simulink model "KD_cl_harness_forthao"  (R2015a)
settings: Solver=ode45  StartTime=0  StopTime=50  FixedStep=0.01  MaxStep=0.005  RelTol=1e-4  AbsTol=1e-4
InitFcn:
  | load KD_const_coeffs_0624
  | load pexhat_stuff
  | load expcon
  | load thr_ff_map
values from neighbouring files (symbols this model uses):
  k1_table = [1 1 1 1 1 1 1 1 1 1 1 1 ... (42 elements, 6x7)]    [thr_ff_map.mat]
  k2_table = [1 1 1 1 1 1 1 1 1 1 1 1 ... (42 elements, 6x7)]    [thr_ff_map.mat]
undefined symbols (not defined in the file or in its folder): c_0, c_1, c_100, c_1000, c_10000, c_1000inv, c_100inv, c_1_int, c_1d2p4, c_1p7, c_4400inv, c_5500inv, c_80, c_90, c_cal_phi, c_compmap, c_ctok, c_fflow_max, c_fflow_min, c_filt, c_flowdiv, c_flowmin, c_flowmult, c_inf, c_km1d2k, c_mm3tokgpers, c_n1, c_p00001, c_p01, c_p016, c_p1429, c_p1e9, c_p4167, c_p4d1p4, c_p5401, c_p9, c_pincomp, c_ra, c_rair, c_Rby1000, c_roacorr, c_rpmtoradpers, c_svrthrottle1, c_svrthrottle2, c_svrthrottlearg, c_svrthrottlebeta, c_ta_max, c_ta_min, c_V, c_vnliftmax, c_vnliftmin, Coefs, const, const_exhat, eegr_map, egrr_delay_init, epim_map, eplufin_ff_map, expcon, invta ... (+15)
libraries: simulink x5
(part 4 of 5)

== system KD_cl_harness_forthao/ctrl_rb_explicit_20131031_v2/expcon/get_ctrl ==
  region : Inport
  u : Inport  Port=2
  calc_u_star : Subsystem
  u_star : Outport
  wires:
  calc_u_star/1(u_star) -> u_star/1
  u/1 -> calc_u_star/2(u)
  region/1 -> calc_u_star/1(region)

== system KD_cl_harness_forthao/ctrl_rb_explicit_20131031_v2/invert_flow/valve_inversion ==
  Ro_a : Inport
  pexhaust : Inport  Port=2
  pintake : Inport  Port=3
  uwegr : Inport  Port=4
  ne_rpm : Inport  Port=5
  Cal_phi1 : Subsystem
  Constant1 : Constant  Value=c_p4167  OutDataTypeStr=single
      settings: AttributesFormatString=%<Value>
  Constant3 : Constant  Value=c_p1429  OutDataTypeStr=single
      settings: AttributesFormatString=%<Value>
  Constant4 : Constant  Value=c_1  OutDataTypeStr=single
      settings: AttributesFormatString=%<Value>
  Constant5 : Constant  Value=c_p5401  OutDataTypeStr=single
      settings: AttributesFormatString=%<Value>
  Pm_by_Pex : Product  Inputs=*/  SaturateOnIntegerOverflow=on  RndMeth=Zero  InputSameDT=on  OutDataTypeStr=Inherit: Same as first input
  Relational Operator : RelationalOperator  Operator=>  OutDataTypeStr=boolean
      settings: AttributesFormatString=%<Operator>
  Saturation1 : Saturate  UpperLimit=c_1  LowerLimit=c_p4167
      settings: AttributesFormatString=%<LowerLimit>\n%<UpperLimit>
  Saturation2 : Saturate  UpperLimit=c_inf  LowerLimit=c_90
      settings: AttributesFormatString=%<LowerLimit>\n%<UpperLimit>
  Saturation3 : Saturate  UpperLimit=c_inf  LowerLimit=c_0
      settings: AttributesFormatString=%<LowerLimit>\n%<UpperLimit>
  Saturation4 : Saturate  UpperLimit=c_inf  LowerLimit=c_p00001
      settings: AttributesFormatString=%<LowerLimit>\n%<UpperLimit>
  Sqrt : Sqrt  AlgorithmType=Newton-Raphson  SaturateOnIntegerOverflow=on
  Sum : Sum  Inputs=|+-
  Sum1 : Sum  Inputs=|++
  Switch2 : Switch  Criteria=u2 ~= 0
      settings: AttributesFormatString=%<Criteria>
  correct flow1 : Product  Inputs=*/  SaturateOnIntegerOverflow=on  RndMeth=Zero  InputSameDT=on  OutDataTypeStr=Inherit: Same as first input
  correct flow2 : Product  Inputs=**  SaturateOnIntegerOverflow=on  RndMeth=Zero  InputSameDT=on  OutDataTypeStr=Inherit: Same as first input
  correct flow3 : Product  Inputs=**  SaturateOnIntegerOverflow=on  RndMeth=Zero  InputSameDT=on  OutDataTypeStr=Inherit: Same as first input
  correct flow4 : Product  Inputs=**  SaturateOnIntegerOverflow=on  RndMeth=Zero  InputSameDT=on  OutDataTypeStr=Inherit: Same as first input
  invert_svr_lut : Lookup2D  RowIndex=invtacols  ColumnIndex=invtarows  Table=invta  LookUpMeth=Interpolation-Use End Values
      settings: AttributesFormatString=%<LookUpMeth>\n%<RowIndex>\n%<ColumnIndex>
  togps : Gain  Gain=c_1000
      settings: AttributesFormatString=%<Gain>
  valve_angle : Outport
  wires:
  Sqrt/1 -> Switch2/1
  correct flow3/1 -> Saturation3/1
  correct flow2/1 -> Sum1/1
  Constant3/1 -> correct flow2/2
  Sum/1 -> correct flow2/1, correct flow3/1
  Constant4/1 -> Sum/1
  invert_svr_lut/1 -> valve_angle/1
  uwegr/1 -> togps/1
  Ro_a/1 -> Cal_phi1/2(Ro_a)
  pexhaust/1 -> [Pex], Saturation2/1
  pintake/1 -> Pm_by_Pex/1
  Pm_by_Pex/1 -> Saturation1/1, Relational Operator/1
  Saturation1/1 -> Sum1/2, Sum/2
  [Pex] -> Cal_phi1/1(Pa)
  Sum1/1 -> correct flow3/2
  Saturation2/1 -> Pm_by_Pex/2
  Saturation3/1 -> Sqrt/1
  Saturation4/1 -> correct flow1/2
  correct flow4/1 -> Saturation4/1
  Switch2/1 -> correct flow4/2
  Cal_phi1/1(phi) -> correct flow4/1
  togps/1 -> correct flow1/1
  Relational Operator/1 -> Switch2/2
  Constant5/1 -> Switch2/3
  Constant1/1 -> Relational Operator/2
  correct flow1/1 -> invert_svr_lut/2
  ne_rpm/1 -> invert_svr_lut/1

== system KD_cl_harness_forthao/ctrl_rb_explicit_20131031_v2/ntestimator/Throttle_Model ==
  TA_deg : Inport
  Ne_rpm : Inport  Port=2
  Pim_Pa : Inport  Port=3
  Tam_K : Inport  Port=4
  wegrthr : Inport  Port=5
  Air_Model_map_use : Subsystem
  Ra : Constant  Value=c_rair  OutDataTypeStr=single  SampleTime=sample_time
      settings: AttributesFormatString=%<Value>\n%<SampleTime>
  p_pre_throttle : Outport  OutDataTypeStr=single
  wires:
  TA_deg/1 -> Air_Model_map_use/1(TA_deg)
  Tam_K/1 -> Air_Model_map_use/4(Ta_K)
  Pim_Pa/1 -> Air_Model_map_use/3(Pim_Pa)
  Ra/1 -> Air_Model_map_use/5(R_a)
  Ne_rpm/1 -> Air_Model_map_use/2(Ne_rpm)
  wegrthr/1 -> Air_Model_map_use/6(wegrthr)
  Air_Model_map_use/1(p_pre_throttle) -> p_pre_throttle/1

== system KD_cl_harness_forthao/ctrl_rb_explicit_20131031_v2/ntestimator/custom_filter ==
  Input : Inport
  Delay1 : Delay  DelayLength=1  InitialCondition=0
  Product1 : Product  Inputs=**  RndMeth=Zero
  Product2 : Product  Inputs=**  RndMeth=Zero
  Saturation1 : Saturate  UpperLimit=1  LowerLimit=0
      settings: AttributesFormatString=%<LowerLimit>\n%<UpperLimit>
  Saturation4 : Saturate  UpperLimit=1  LowerLimit=0
      settings: AttributesFormatString=%<LowerLimit>\n%<UpperLimit>
  Sum1 : Sum  Inputs=+-|
  Sum11 : Sum  Inputs=++|
  filt : Constant  Value=c_filt  OutDataTypeStr=single  SampleTime=sample_time
      settings: AttributesFormatString=%<Value>\n%<SampleTime>
  filt1 : Constant  Value=c_filt  OutDataTypeStr=single  SampleTime=sample_time
      settings: AttributesFormatString=%<Value>\n%<SampleTime>
  one : Constant  OutDataTypeStr=single  SampleTime=sample_time
      settings: AttributesFormatString=%<Value>\n%<SampleTime>
  Output : Outport  OutDataTypeStr=single
  wires:
  Input/1 -> Product1/2
  Delay1/1 -> Product2/1
  filt/1 -> Saturation1/1
  Product2/1 -> Sum11/1
  Sum1/1 -> Product1/1
  filt1/1 -> Saturation4/1
  Saturation4/1 -> Sum1/2
  Saturation1/1 -> Product2/2
  Product1/1 -> Sum11/2
  one/1 -> Sum1/1
  Sum11/1 -> Output/1, Delay1/1

== system KD_cl_harness_forthao/ctrl_rb_explicit_20131031_v2/rpm1200testpattern/IfActionSubsystem ==
  Action Port : ActionPort  ActionType=then
  tp : Constant  Value=[150;50;150]  OutDataTypeStr=single  SampleTime=sample_time
      settings: AttributesFormatString=%<Value>\n%<SampleTime>
  Out1 : Outport  InitialOutput=[150;50;150]
  wires:
  tp/1 -> Out1/1

== system KD_cl_harness_forthao/ctrl_rb_explicit_20131031_v2/rpm1200testpattern/IfActionSubsystem1 ==
  Action Port : ActionPort  ActionType=elseif
  tp : Constant  Value=[150;50;150]  OutDataTypeStr=single  SampleTime=sample_time
      settings: AttributesFormatString=%<Value>\n%<SampleTime>
  Out1 : Outport  InitialOutput=[150;50;150]
  wires:
  tp/1 -> Out1/1

== system KD_cl_harness_forthao/ctrl_rb_explicit_20131031_v2/rpm1200testpattern/IfActionSubsystem10 ==
  Action Port : ActionPort  ActionType=elseif
  tp : Constant  Value=[150;50;150]  OutDataTypeStr=single  SampleTime=sample_time
      settings: AttributesFormatString=%<Value>\n%<SampleTime>
  Out1 : Outport  InitialOutput=[150;50;150]
  wires:
  tp/1 -> Out1/1

== system KD_cl_harness_forthao/ctrl_rb_explicit_20131031_v2/rpm1200testpattern/IfActionSubsystem11 ==
  Action Port : ActionPort  ActionType=elseif
  tp : Constant  Value=[150;50;150]  OutDataTypeStr=single  SampleTime=sample_time
      settings: AttributesFormatString=%<Value>\n%<SampleTime>
  Out1 : Outport  InitialOutput=[150;50;150]
  wires:
  tp/1 -> Out1/1

== system KD_cl_harness_forthao/ctrl_rb_explicit_20131031_v2/rpm1200testpattern/IfActionSubsystem12 ==
  Action Port : ActionPort  ActionType=elseif
  tp : Constant  Value=[150;50;150]  OutDataTypeStr=single  SampleTime=sample_time
      settings: AttributesFormatString=%<Value>\n%<SampleTime>
  Out1 : Outport  InitialOutput=[150;50;150]
  wires:
  tp/1 -> Out1/1

== system KD_cl_harness_forthao/ctrl_rb_explicit_20131031_v2/rpm1200testpattern/IfActionSubsystem13 ==
  Action Port : ActionPort  ActionType=elseif
  tp : Constant  Value=[150;50;150]  OutDataTypeStr=single  SampleTime=sample_time
      settings: AttributesFormatString=%<Value>\n%<SampleTime>
  Out1 : Outport  InitialOutput=[150;50;150]
  wires:
  tp/1 -> Out1/1

== system KD_cl_harness_forthao/ctrl_rb_explicit_20131031_v2/rpm1200testpattern/IfActionSubsystem14 ==
  Action Port : ActionPort  ActionType=elseif
  tp : Constant  Value=[150;50;150]  OutDataTypeStr=single  SampleTime=sample_time
      settings: AttributesFormatString=%<Value>\n%<SampleTime>
  Out1 : Outport  InitialOutput=[150;50;150]
  wires:
  tp/1 -> Out1/1

== system KD_cl_harness_forthao/ctrl_rb_explicit_20131031_v2/rpm1200testpattern/IfActionSubsystem15 ==
  Action Port : ActionPort  ActionType=elseif
  tp : Constant  Value=[150;20;150]  OutDataTypeStr=single  SampleTime=sample_time
      settings: AttributesFormatString=%<Value>\n%<SampleTime>
  Out1 : Outport  InitialOutput=[150;20;150]
  wires:
  tp/1 -> Out1/1

== system KD_cl_harness_forthao/ctrl_rb_explicit_20131031_v2/rpm1200testpattern/IfActionSubsystem16 ==
  Action Port : ActionPort  ActionType=elseif
  tp : Constant  Value=[150;5;150]  OutDataTypeStr=single  SampleTime=sample_time
      settings: AttributesFormatString=%<Value>\n%<SampleTime>
  Out1 : Outport  InitialOutput=[150;5;150]
  wires:
  tp/1 -> Out1/1

== system KD_cl_harness_forthao/ctrl_rb_explicit_20131031_v2/rpm1200testpattern/IfActionSubsystem17 ==
  Action Port : ActionPort  ActionType=elseif
  tp : Constant  Value=[150;15;150]  OutDataTypeStr=single  SampleTime=sample_time
      settings: AttributesFormatString=%<Value>\n%<SampleTime>
  Out1 : Outport  InitialOutput=[150;15;150]
  wires:
  tp/1 -> Out1/1

== system KD_cl_harness_forthao/ctrl_rb_explicit_20131031_v2/rpm1200testpattern/IfActionSubsystem18 ==
  Action Port : ActionPort  ActionType=elseif
  tp : Constant  Value=[130;20;150]  OutDataTypeStr=single  SampleTime=sample_time
      settings: AttributesFormatString=%<Value>\n%<SampleTime>
  Out1 : Outport  InitialOutput=[130;20;150]
  wires:
  tp/1 -> Out1/1

== system KD_cl_harness_forthao/ctrl_rb_explicit_20131031_v2/rpm1200testpattern/IfActionSubsystem19 ==
  Action Port : ActionPort  ActionType=elseif
  tp : Constant  Value=[130;20;115]  OutDataTypeStr=single  SampleTime=sample_time
      settings: AttributesFormatString=%<Value>\n%<SampleTime>
  Out1 : Outport  InitialOutput=[130;20;115]
  wires:
  tp/1 -> Out1/1

== system KD_cl_harness_forthao/ctrl_rb_explicit_20131031_v2/rpm1200testpattern/IfActionSubsystem2 ==
  Action Port : ActionPort  ActionType=elseif
  tp : Constant  Value=[150;50;150]  OutDataTypeStr=single  SampleTime=sample_time
      settings: AttributesFormatString=%<Value>\n%<SampleTime>
  Out1 : Outport  InitialOutput=[150;50;150]
  wires:
  tp/1 -> Out1/1

== system KD_cl_harness_forthao/ctrl_rb_explicit_20131031_v2/rpm1200testpattern/IfActionSubsystem20 ==
  Action Port : ActionPort  ActionType=elseif
  tp : Constant  Value=[130;20;110]  OutDataTypeStr=single  SampleTime=sample_time
      settings: AttributesFormatString=%<Value>\n%<SampleTime>
  Out1 : Outport  InitialOutput=[130;20;110]
  wires:
  tp/1 -> Out1/1

== system KD_cl_harness_forthao/ctrl_rb_explicit_20131031_v2/rpm1200testpattern/IfActionSubsystem21 ==
  Action Port : ActionPort  ActionType=elseif
  tp : Constant  Value=[130;20;105]  OutDataTypeStr=single  SampleTime=sample_time
      settings: AttributesFormatString=%<Value>\n%<SampleTime>
  Out1 : Outport  InitialOutput=[130;20;105]
  wires:
  tp/1 -> Out1/1

== system KD_cl_harness_forthao/ctrl_rb_explicit_20131031_v2/rpm1200testpattern/IfActionSubsystem22 ==
  Action Port : ActionPort  ActionType=elseif
  tp : Constant  Value=[130;0;105]  OutDataTypeStr=single  SampleTime=sample_time
      settings: AttributesFormatString=%<Value>\n%<SampleTime>
  Out1 : Outport  InitialOutput=[130;0;105]
  wires:
  tp/1 -> Out1/1

== system KD_cl_harness_forthao/ctrl_rb_explicit_20131031_v2/rpm1200testpattern/IfActionSubsystem23 ==
  Action Port : ActionPort  ActionType=elseif
  tp : Constant  Value=[130;0;110]  OutDataTypeStr=single  SampleTime=sample_time
      settings: AttributesFormatString=%<Value>\n%<SampleTime>
  Out1 : Outport  InitialOutput=[130;0;110]
  wires:
  tp/1 -> Out1/1

== system KD_cl_harness_forthao/ctrl_rb_explicit_20131031_v2/rpm1200testpattern/IfActionSubsystem24 ==
  Action Port : ActionPort  ActionType=elseif
  tp : Constant  Value=[150;3;150]  OutDataTypeStr=single  SampleTime=sample_time
      settings: AttributesFormatString=%<Value>\n%<SampleTime>
  Out1 : Outport  InitialOutput=[150;3;150]
  wires:
  tp/1 -> Out1/1

== system KD_cl_harness_forthao/ctrl_rb_explicit_20131031_v2/rpm1200testpattern/IfActionSubsystem25 ==
  Action Port : ActionPort  ActionType=elseif
  tp : Constant  Value=[150;10;150]  OutDataTypeStr=single  SampleTime=sample_time
      settings: AttributesFormatString=%<Value>\n%<SampleTime>
  Out1 : Outport  InitialOutput=[150;10;150]
  wires:
  tp/1 -> Out1/1

== system KD_cl_harness_forthao/ctrl_rb_explicit_20131031_v2/rpm1200testpattern/IfActionSubsystem26 ==
  Action Port : ActionPort  ActionType=elseif
  tp : Constant  Value=[150;20;150]  OutDataTypeStr=single  SampleTime=sample_time
      settings: AttributesFormatString=%<Value>\n%<SampleTime>
  Out1 : Outport  InitialOutput=[150;20;150]
  wires:
  tp/1 -> Out1/1

== system KD_cl_harness_forthao/ctrl_rb_explicit_20131031_v2/rpm1200testpattern/IfActionSubsystem27 ==
  Action Port : ActionPort  ActionType=elseif
  tp : Constant  Value=[150;20;150]  OutDataTypeStr=single  SampleTime=sample_time
      settings: AttributesFormatString=%<Value>\n%<SampleTime>
  Out1 : Outport  InitialOutput=[150;20;150]
  wires:
  tp/1 -> Out1/1

== system KD_cl_harness_forthao/ctrl_rb_explicit_20131031_v2/rpm1200testpattern/IfActionSubsystem28 ==
  Action Port : ActionPort  ActionType=elseif
  tp : Constant  Value=[110;20;150]  OutDataTypeStr=single  SampleTime=sample_time
      settings: AttributesFormatString=%<Value>\n%<SampleTime>
  Out1 : Outport  InitialOutput=[110;20;150]
  wires:
  tp/1 -> Out1/1

== system KD_cl_harness_forthao/ctrl_rb_explicit_20131031_v2/rpm1200testpattern/IfActionSubsystem29 ==
  Action Port : ActionPort  ActionType=elseif
  tp : Constant  Value=[100;20;150]  OutDataTypeStr=single  SampleTime=sample_time
      settings: AttributesFormatString=%<Value>\n%<SampleTime>
  Out1 : Outport  InitialOutput=[100;20;150]
  wires:
  tp/1 -> Out1/1

== system KD_cl_harness_forthao/ctrl_rb_explicit_20131031_v2/rpm1200testpattern/IfActionSubsystem3 ==
  Action Port : ActionPort  ActionType=elseif
  tp : Constant  Value=[150;50;150]  OutDataTypeStr=single  SampleTime=sample_time
      settings: AttributesFormatString=%<Value>\n%<SampleTime>
  Out1 : Outport  InitialOutput=[150;50;150]
  wires:
  tp/1 -> Out1/1

== system KD_cl_harness_forthao/ctrl_rb_explicit_20131031_v2/rpm1200testpattern/IfActionSubsystem30 ==
  Action Port : ActionPort  ActionType=elseif
  tp : Constant  Value=[115;20;150]  OutDataTypeStr=single  SampleTime=sample_time
      settings: AttributesFormatString=%<Value>\n%<SampleTime>
  Out1 : Outport  InitialOutput=[115;20;150]
  wires:
  tp/1 -> Out1/1

== system KD_cl_harness_forthao/ctrl_rb_explicit_20131031_v2/rpm1200testpattern/IfActionSubsystem31 ==
  Action Port : ActionPort  ActionType=elseif
  tp : Constant  Value=[105;20;150]  OutDataTypeStr=single  SampleTime=sample_time
      settings: AttributesFormatString=%<Value>\n%<SampleTime>
  Out1 : Outport  InitialOutput=[105;20;150]
  wires:
  tp/1 -> Out1/1

== system KD_cl_harness_forthao/ctrl_rb_explicit_20131031_v2/rpm1200testpattern/IfActionSubsystem32 ==
  Action Port : ActionPort  ActionType=elseif
  tp : Constant  Value=[105;0;110]  OutDataTypeStr=single  SampleTime=sample_time
      settings: AttributesFormatString=%<Value>\n%<SampleTime>
  Out1 : Outport  InitialOutput=[105;0;110]
  wires:
  tp/1 -> Out1/1

== system KD_cl_harness_forthao/ctrl_rb_explicit_20131031_v2/rpm1200testpattern/IfActionSubsystem33 ==
  Action Port : ActionPort  ActionType=elseif
  tp : Constant  Value=[100;0;110]  OutDataTypeStr=single  SampleTime=sample_time
      settings: AttributesFormatString=%<Value>\n%<SampleTime>
  Out1 : Outport  InitialOutput=[100;0;110]
  wires:
  tp/1 -> Out1/1

== system KD_cl_harness_forthao/ctrl_rb_explicit_20131031_v2/rpm1200testpattern/IfActionSubsystem34 ==
  Action Port : ActionPort  ActionType=else
  tp : Constant  Value=[150;50;150]  OutDataTypeStr=single  SampleTime=sample_time
      settings: AttributesFormatString=%<Value>\n%<SampleTime>
  Out1 : Outport  InitialOutput=[150;50;150]
  wires:
  tp/1 -> Out1/1

== system KD_cl_harness_forthao/ctrl_rb_explicit_20131031_v2/rpm1200testpattern/IfActionSubsystem4 ==
  Action Port : ActionPort  ActionType=elseif
  tp : Constant  Value=[150;50;150]  OutDataTypeStr=single  SampleTime=sample_time
      settings: AttributesFormatString=%<Value>\n%<SampleTime>
  Out1 : Outport  InitialOutput=[150;50;150]
  wires:
  tp/1 -> Out1/1

== system KD_cl_harness_forthao/ctrl_rb_explicit_20131031_v2/rpm1200testpattern/IfActionSubsystem5 ==
  Action Port : ActionPort  ActionType=elseif
  tp : Constant  Value=[150;50;150]  OutDataTypeStr=single  SampleTime=sample_time
      settings: AttributesFormatString=%<Value>\n%<SampleTime>
  Out1 : Outport  InitialOutput=[150;50;150]
  wires:
  tp/1 -> Out1/1

== system KD_cl_harness_forthao/ctrl_rb_explicit_20131031_v2/rpm1200testpattern/IfActionSubsystem6 ==
  Action Port : ActionPort  ActionType=elseif
  tp : Constant  Value=[150;50;150]  OutDataTypeStr=single  SampleTime=sample_time
      settings: AttributesFormatString=%<Value>\n%<SampleTime>
  Out1 : Outport  InitialOutput=[150;50;150]
  wires:
  tp/1 -> Out1/1

== system KD_cl_harness_forthao/ctrl_rb_explicit_20131031_v2/rpm1200testpattern/IfActionSubsystem7 ==
  Action Port : ActionPort  ActionType=elseif
  tp : Constant  Value=[150;50;150]  OutDataTypeStr=single  SampleTime=sample_time
      settings: AttributesFormatString=%<Value>\n%<SampleTime>
  Out1 : Outport  InitialOutput=[150;50;150]
  wires:
  tp/1 -> Out1/1

== system KD_cl_harness_forthao/ctrl_rb_explicit_20131031_v2/rpm1200testpattern/IfActionSubsystem8 ==
  Action Port : ActionPort  ActionType=elseif
  tp : Constant  Value=[150;50;150]  OutDataTypeStr=single  SampleTime=sample_time
      settings: AttributesFormatString=%<Value>\n%<SampleTime>
  Out1 : Outport  InitialOutput=[150;50;150]
  wires:
  tp/1 -> Out1/1

== system KD_cl_harness_forthao/ctrl_rb_explicit_20131031_v2/rpm1200testpattern/IfActionSubsystem9 ==
  Action Port : ActionPort  ActionType=elseif
  tp : Constant  Value=[150;50;150]  OutDataTypeStr=single  SampleTime=sample_time
      settings: AttributesFormatString=%<Value>\n%<SampleTime>
  Out1 : Outport  InitialOutput=[150;50;150]
  wires:
  tp/1 -> Out1/1

== system KD_cl_harness_forthao/ctrl_rb_explicit_20131031_v2/rpm2500testpattern/IfActionSubsystem ==
  Action Port : ActionPort  ActionType=then
  tp : Constant  Value=[170;50;250]  OutDataTypeStr=single  SampleTime=sample_time
      settings: AttributesFormatString=%<Value>\n%<SampleTime>
  Out1 : Outport  InitialOutput=[170;50;250]
  wires:
  tp/1 -> Out1/1

== system KD_cl_harness_forthao/ctrl_rb_explicit_20131031_v2/rpm2500testpattern/IfActionSubsystem1 ==
  Action Port : ActionPort  ActionType=elseif
  tp : Constant  Value=[170;50;250]  OutDataTypeStr=single  SampleTime=sample_time
      settings: AttributesFormatString=%<Value>\n%<SampleTime>
  Out1 : Outport  InitialOutput=[170;50;250]
  wires:
  tp/1 -> Out1/1

== system KD_cl_harness_forthao/ctrl_rb_explicit_20131031_v2/rpm2500testpattern/IfActionSubsystem10 ==
  Action Port : ActionPort  ActionType=elseif
  tp : Constant  Value=[160;50;250]  OutDataTypeStr=single  SampleTime=sample_time
      settings: AttributesFormatString=%<Value>\n%<SampleTime>
  Out1 : Outport  InitialOutput=[160;50;250]
  wires:
  tp/1 -> Out1/1

== system KD_cl_harness_forthao/ctrl_rb_explicit_20131031_v2/rpm2500testpattern/IfActionSubsystem11 ==
  Action Port : ActionPort  ActionType=elseif
  tp : Constant  Value=[160;0;250]  OutDataTypeStr=single  SampleTime=sample_time
      settings: AttributesFormatString=%<Value>\n%<SampleTime>
  Out1 : Outport  InitialOutput=[160;0;250]
  wires:
  tp/1 -> Out1/1

== system KD_cl_harness_forthao/ctrl_rb_explicit_20131031_v2/rpm2500testpattern/IfActionSubsystem12 ==
  Action Port : ActionPort  ActionType=elseif
  tp : Constant  Value=[160;15;250]  OutDataTypeStr=single  SampleTime=sample_time
      settings: AttributesFormatString=%<Value>\n%<SampleTime>
  Out1 : Outport  InitialOutput=[160;15;250]
  wires:
  tp/1 -> Out1/1

== system KD_cl_harness_forthao/ctrl_rb_explicit_20131031_v2/rpm2500testpattern/IfActionSubsystem13 ==
  Action Port : ActionPort  ActionType=elseif
  tp : Constant  Value=[160;3;250]  OutDataTypeStr=single  SampleTime=sample_time
      settings: AttributesFormatString=%<Value>\n%<SampleTime>
  Out1 : Outport  InitialOutput=[160;3;250]
  wires:
  tp/1 -> Out1/1

== system KD_cl_harness_forthao/ctrl_rb_explicit_20131031_v2/rpm2500testpattern/IfActionSubsystem14 ==
  Action Port : ActionPort  ActionType=elseif
  tp : Constant  Value=[150;3;250]  OutDataTypeStr=single  SampleTime=sample_time
      settings: AttributesFormatString=%<Value>\n%<SampleTime>
  Out1 : Outport  InitialOutput=[150;3;250]
  wires:
  tp/1 -> Out1/1

== system KD_cl_harness_forthao/ctrl_rb_explicit_20131031_v2/rpm2500testpattern/IfActionSubsystem15 ==
  Action Port : ActionPort  ActionType=elseif
  tp : Constant  Value=[140;3;250]  OutDataTypeStr=single  SampleTime=sample_time
      settings: AttributesFormatString=%<Value>\n%<SampleTime>
  Out1 : Outport  InitialOutput=[140;3;250]
  wires:
  tp/1 -> Out1/1

== system KD_cl_harness_forthao/ctrl_rb_explicit_20131031_v2/rpm2500testpattern/IfActionSubsystem16 ==
  Action Port : ActionPort  ActionType=elseif
  tp : Constant  Value=[140;0;250]  OutDataTypeStr=single  SampleTime=sample_time
      settings: AttributesFormatString=%<Value>\n%<SampleTime>
  Out1 : Outport  InitialOutput=[140;0;250]
  wires:
  tp/1 -> Out1/1

== system KD_cl_harness_forthao/ctrl_rb_explicit_20131031_v2/rpm2500testpattern/IfActionSubsystem17 ==
  Action Port : ActionPort  ActionType=elseif
  tp : Constant  Value=[140;20;250]  OutDataTypeStr=single  SampleTime=sample_time
      settings: AttributesFormatString=%<Value>\n%<SampleTime>
  Out1 : Outport  InitialOutput=[140;20;250]
  wires:
  tp/1 -> Out1/1

== system KD_cl_harness_forthao/ctrl_rb_explicit_20131031_v2/rpm2500testpattern/IfActionSubsystem18 ==
  Action Port : ActionPort  ActionType=elseif
  tp : Constant  Value=[140;0;110]  OutDataTypeStr=single  SampleTime=sample_time
      settings: AttributesFormatString=%<Value>\n%<SampleTime>
  Out1 : Outport  InitialOutput=[140;0;110]
  wires:
  tp/1 -> Out1/1

== system KD_cl_harness_forthao/ctrl_rb_explicit_20131031_v2/rpm2500testpattern/IfActionSubsystem19 ==
  Action Port : ActionPort  ActionType=elseif
  tp : Constant  Value=[140;10;110]  OutDataTypeStr=single  SampleTime=sample_time
      settings: AttributesFormatString=%<Value>\n%<SampleTime>
  Out1 : Outport  InitialOutput=[140;10;110]
  wires:
  tp/1 -> Out1/1

== system KD_cl_harness_forthao/ctrl_rb_explicit_20131031_v2/rpm2500testpattern/IfActionSubsystem2 ==
  Action Port : ActionPort  ActionType=elseif
  tp : Constant  Value=[170;50;250]  OutDataTypeStr=single  SampleTime=sample_time
      settings: AttributesFormatString=%<Value>\n%<SampleTime>
  Out1 : Outport  InitialOutput=[170;50;250]
  wires:
  tp/1 -> Out1/1

== system KD_cl_harness_forthao/ctrl_rb_explicit_20131031_v2/rpm2500testpattern/IfActionSubsystem20 ==
  Action Port : ActionPort  ActionType=elseif
  tp : Constant  Value=[140;10;120]  OutDataTypeStr=single  SampleTime=sample_time
      settings: AttributesFormatString=%<Value>\n%<SampleTime>
  Out1 : Outport  InitialOutput=[140;10;120]
  wires:
  tp/1 -> Out1/1

== system KD_cl_harness_forthao/ctrl_rb_explicit_20131031_v2/rpm2500testpattern/IfActionSubsystem21 ==
  Action Port : ActionPort  ActionType=elseif
  tp : Constant  Value=[140;10;150]  OutDataTypeStr=single  SampleTime=sample_time
      settings: AttributesFormatString=%<Value>\n%<SampleTime>
  Out1 : Outport  InitialOutput=[140;10;150]
  wires:
  tp/1 -> Out1/1

== system KD_cl_harness_forthao/ctrl_rb_explicit_20131031_v2/rpm2500testpattern/IfActionSubsystem22 ==
  Action Port : ActionPort  ActionType=elseif
  tp : Constant  Value=[140;10;110]  OutDataTypeStr=single  SampleTime=sample_time
      settings: AttributesFormatString=%<Value>\n%<SampleTime>
  Out1 : Outport  InitialOutput=[140;10;110]
  wires:
  tp/1 -> Out1/1

== system KD_cl_harness_forthao/ctrl_rb_explicit_20131031_v2/rpm2500testpattern/IfActionSubsystem23 ==
  Action Port : ActionPort  ActionType=elseif
  tp : Constant  Value=[140;10;150]  OutDataTypeStr=single  SampleTime=sample_time
      settings: AttributesFormatString=%<Value>\n%<SampleTime>
  Out1 : Outport  InitialOutput=[140;10;150]
  wires:
  tp/1 -> Out1/1

== system KD_cl_harness_forthao/ctrl_rb_explicit_20131031_v2/rpm2500testpattern/IfActionSubsystem24 ==
  Action Port : ActionPort  ActionType=elseif
  tp : Constant  Value=[140;20;250]  OutDataTypeStr=single  SampleTime=sample_time
      settings: AttributesFormatString=%<Value>\n%<SampleTime>
  Out1 : Outport  InitialOutput=[140;20;250]
  wires:
  tp/1 -> Out1/1

== system KD_cl_harness_forthao/ctrl_rb_explicit_20131031_v2/rpm2500testpattern/IfActionSubsystem25 ==
  Action Port : ActionPort  ActionType=elseif
  tp : Constant  Value=[140;20;250]  OutDataTypeStr=single  SampleTime=sample_time
      settings: AttributesFormatString=%<Value>\n%<SampleTime>
  Out1 : Outport  InitialOutput=[140;20;250]
  wires:
  tp/1 -> Out1/1

== system KD_cl_harness_forthao/ctrl_rb_explicit_20131031_v2/rpm2500testpattern/IfActionSubsystem26 ==
  Action Port : ActionPort  ActionType=elseif
  tp : Constant  Value=[140;20;250]  OutDataTypeStr=single  SampleTime=sample_time
      settings: AttributesFormatString=%<Value>\n%<SampleTime>
  Out1 : Outport  InitialOutput=[140;20;250]
  wires:
  tp/1 -> Out1/1

== system KD_cl_harness_forthao/ctrl_rb_explicit_20131031_v2/rpm2500testpattern/IfActionSubsystem27 ==
  Action Port : ActionPort  ActionType=elseif
  tp : Constant  Value=[140;20;250]  OutDataTypeStr=single  SampleTime=sample_time
      settings: AttributesFormatString=%<Value>\n%<SampleTime>
  Out1 : Outport  InitialOutput=[140;20;250]
  wires:
  tp/1 -> Out1/1

== system KD_cl_harness_forthao/ctrl_rb_explicit_20131031_v2/rpm2500testpattern/IfActionSubsystem28 ==
  Action Port : ActionPort  ActionType=elseif
  tp : Constant  Value=[140;20;250]  OutDataTypeStr=single  SampleTime=sample_time
      settings: AttributesFormatString=%<Value>\n%<SampleTime>
  Out1 : Outport  InitialOutput=[140;20;250]
  wires:
  tp/1 -> Out1/1

== system KD_cl_harness_forthao/ctrl_rb_explicit_20131031_v2/rpm2500testpattern/IfActionSubsystem29 ==
  Action Port : ActionPort  ActionType=elseif
  tp : Constant  Value=[140;20;125]  OutDataTypeStr=single  SampleTime=sample_time
      settings: AttributesFormatString=%<Value>\n%<SampleTime>
  Out1 : Outport  InitialOutput=[140;20;125]
  wires:
  tp/1 -> Out1/1

== system KD_cl_harness_forthao/ctrl_rb_explicit_20131031_v2/rpm2500testpattern/IfActionSubsystem3 ==
  Action Port : ActionPort  ActionType=elseif
  tp : Constant  Value=[158;50;250]  OutDataTypeStr=single  SampleTime=sample_time
      settings: AttributesFormatString=%<Value>\n%<SampleTime>
  Out1 : Outport  InitialOutput=[158;50;250]
  wires:
  tp/1 -> Out1/1

== system KD_cl_harness_forthao/ctrl_rb_explicit_20131031_v2/rpm2500testpattern/IfActionSubsystem30 ==
  Action Port : ActionPort  ActionType=elseif
  tp : Constant  Value=[140;20;120]  OutDataTypeStr=single  SampleTime=sample_time
      settings: AttributesFormatString=%<Value>\n%<SampleTime>
  Out1 : Outport  InitialOutput=[140;20;120]
  wires:
  tp/1 -> Out1/1

== system KD_cl_harness_forthao/ctrl_rb_explicit_20131031_v2/rpm2500testpattern/IfActionSubsystem31 ==
  Action Port : ActionPort  ActionType=elseif
  tp : Constant  Value=[140;20;110]  OutDataTypeStr=single  SampleTime=sample_time
      settings: AttributesFormatString=%<Value>\n%<SampleTime>
  Out1 : Outport  InitialOutput=[140;20;110]
  wires:
  tp/1 -> Out1/1

== system KD_cl_harness_forthao/ctrl_rb_explicit_20131031_v2/rpm2500testpattern/IfActionSubsystem32 ==
  Action Port : ActionPort  ActionType=else
  tp : Constant  Value=[170;50;250]  OutDataTypeStr=single  SampleTime=sample_time
      settings: AttributesFormatString=%<Value>\n%<SampleTime>
  Out1 : Outport  InitialOutput=[170;50;250]
  wires:
  tp/1 -> Out1/1

== system KD_cl_harness_forthao/ctrl_rb_explicit_20131031_v2/rpm2500testpattern/IfActionSubsystem4 ==
  Action Port : ActionPort  ActionType=elseif
  tp : Constant  Value=[158;50;250]  OutDataTypeStr=single  SampleTime=sample_time
      settings: AttributesFormatString=%<Value>\n%<SampleTime>
  Out1 : Outport  InitialOutput=[158;50;250]
  wires:
  tp/1 -> Out1/1

== system KD_cl_harness_forthao/ctrl_rb_explicit_20131031_v2/rpm2500testpattern/IfActionSubsystem5 ==
  Action Port : ActionPort  ActionType=elseif
  tp : Constant  Value=[158;50;250]  OutDataTypeStr=single  SampleTime=sample_time
      settings: AttributesFormatString=%<Value>\n%<SampleTime>
  Out1 : Outport  InitialOutput=[158;50;250]
  wires:
  tp/1 -> Out1/1

== system KD_cl_harness_forthao/ctrl_rb_explicit_20131031_v2/rpm2500testpattern/IfActionSubsystem6 ==
  Action Port : ActionPort  ActionType=elseif
  tp : Constant  Value=[158;50;250]  OutDataTypeStr=single  SampleTime=sample_time
      settings: AttributesFormatString=%<Value>\n%<SampleTime>
  Out1 : Outport  InitialOutput=[158;50;250]
  wires:
  tp/1 -> Out1/1

== system KD_cl_harness_forthao/ctrl_rb_explicit_20131031_v2/rpm2500testpattern/IfActionSubsystem7 ==
  Action Port : ActionPort  ActionType=elseif
  tp : Constant  Value=[150;50;250]  OutDataTypeStr=single  SampleTime=sample_time
      settings: AttributesFormatString=%<Value>\n%<SampleTime>
  Out1 : Outport  InitialOutput=[150;50;250]
  wires:
  tp/1 -> Out1/1

== system KD_cl_harness_forthao/ctrl_rb_explicit_20131031_v2/rpm2500testpattern/IfActionSubsystem8 ==
  Action Port : ActionPort  ActionType=elseif
  tp : Constant  Value=[170;50;250]  OutDataTypeStr=single  SampleTime=sample_time
      settings: AttributesFormatString=%<Value>\n%<SampleTime>
  Out1 : Outport  InitialOutput=[170;50;250]
  wires:
  tp/1 -> Out1/1

== system KD_cl_harness_forthao/ctrl_rb_explicit_20131031_v2/rpm2500testpattern/IfActionSubsystem9 ==
  Action Port : ActionPort  ActionType=elseif
  tp : Constant  Value=[140;50;250]  OutDataTypeStr=single  SampleTime=sample_time
      settings: AttributesFormatString=%<Value>\n%<SampleTime>
  Out1 : Outport  InitialOutput=[140;50;250]
  wires:
  tp/1 -> Out1/1

== system KD_cl_harness_forthao/ctrl_rb_explicit_20131031_v2/set_point_maps/EGR_rate_map ==
  fuel_rate_mm3perst : Inport
  engine_speed : Inport  Port=2
  Gain2 : Gain  Gain=c_100
      settings: AttributesFormatString=%<Gain>
  epimbs_map : Lookup2D  RowIndex=eegr_map.x  ColumnIndex=eegr_map.y  Table=eegr_map.z  LookUpMeth=Interpolation-Use End Values
      settings: AttributesFormatString=%<LookUpMeth>\n%<RowIndex>\n%<ColumnIndex>
  EGR_rate_ref : Outport
  wires:
  epimbs_map/1 -> Gain2/1
  Gain2/1 -> EGR_rate_ref/1
  fuel_rate_mm3perst/1 -> epimbs_map/2
  engine_speed/1 -> epimbs_map/1

== system KD_cl_harness_forthao/ctrl_rb_explicit_20131031_v2/set_point_maps/intake_pressure_map ==
  fuel_rate_mm3perst : Inport
  engine_speed : Inport  Port=2
  boost_pressure_map : Subsystem
  intake_manifold_pressure_ref : Outport
  wires:
  engine_speed/1 -> boost_pressure_map/2(engine_speed)
  fuel_rate_mm3perst/1 -> boost_pressure_map/1(fuel_rate_mm3perst)
  boost_pressure_map/1(intake_manifold_pressure) -> intake_manifold_pressure_ref/1

== system KD_cl_harness_forthao/pre-throttle manifold/p_preThrottle/Cus_integrator ==
  in : Inport
  p_prethrottle (kPa)1 : Integrator  InitialCondition=IV.p_prethrottle  UpperSaturationLimit=maxL.p_PreThrottle  LowerSaturationLimit=minL.p_PreThrottle
  p_preThrottle : Outport
  wires:
  p_prethrottle (kPa)1/1 -> p_preThrottle/1
  in/1 -> p_prethrottle (kPa)1/1

== system KD_cl_harness_forthao/EGR Throttle/EGR Throttle/Throttle Model2/Air Model_map_use ==
  TA[deg] : Inport
  Ne[rpm] : Inport  Port=2
  Pim[Pa] : Inport  Port=3
  Tim[K] : Inport  Port=4
  Pa[Pa] : Inport  Port=5
  Ta[K] : Inport  Port=6
  R_im : Inport  Port=7
  R_a : Inport  Port=8
  Back-Flow : Subsystem
  Forward-Flow : Subsystem
  Gain : Gain  Gain=-1
  Product : Product  Inputs=/*  SaturateOnIntegerOverflow=on  RndMeth=Zero  InputSameDT=on  OutDataTypeStr=Inherit: Same as first input
  Product1 : Product  Inputs=*//  SaturateOnIntegerOverflow=on  RndMeth=Zero  InputSameDT=on  OutDataTypeStr=Inherit: Same as first input
  Product3 : Product  Inputs=*//  SaturateOnIntegerOverflow=on  RndMeth=Zero  InputSameDT=on  OutDataTypeStr=Inherit: Same as first input
  Switch : Switch  Threshold=1  SaturateOnIntegerOverflow=on  InputSameDT=on
  mt[kg/sec] : Outport
  forwardmt : Outport  Port=2
  backwardmt : Outport  Port=3
  wires:
  Product1/1 -> Forward-Flow/1(Ro_a)
  Switch/1 -> mt[kg/sec]/1
  Product/1 -> Switch/2
  TA[deg]/1 -> Forward-Flow/2(TA[deg]), Back-Flow/1(TA[deg])
  [Pa] -> Product/2, Forward-Flow/4(Pa), Back-Flow/4(Pa)
  Pim[Pa]/1 -> Forward-Flow/5(Pm), Product/1, Back-Flow/5(Pm), Product3/1
  Pa[Pa]/1 -> [Pa]
  Ta[K]/1 -> [Ta]
  R_a/1 -> [Ra]
  R_im/1 -> [Rim]
  [Ra] -> Product1/3
  [Pa] -> Product1/1
  [Ta] -> Product1/2
  [Rim] -> Product3/3
  Tim[K]/1 -> Product3/2
  Forward-Flow/1(mt_dot[kg/s]) -> Switch/1, forwardmt/1
  Product3/1 -> Back-Flow/3(Ro_m)
  Back-Flow/1(mt_dot[kg/s]) -> Gain/1
  Ne[rpm]/1 -> Forward-Flow/3(Ne[rpm]), Back-Flow/2(Ne[rpm])
  Gain/1 -> Switch/3, backwardmt/1

== system KD_cl_harness_forthao/EGR Valve/SVR EGR/EGR_model/Air Model_map_use ==
  TA[deg] : Inport
  Ne[rpm] : Inport  Port=2
  Pim[Pa] : Inport  Port=3
  Tim[K] : Inport  Port=4
  Pa[Pa] : Inport  Port=5
  Ta[K] : Inport  Port=6
  R_im : Inport  Port=7
  R_a : Inport  Port=8
  Back-Flow : Subsystem
  Forward-Flow : Subsystem
  Gain : Gain  Gain=-1
  Product : Product  Inputs=/*  SaturateOnIntegerOverflow=on  RndMeth=Zero  InputSameDT=on  OutDataTypeStr=Inherit: Same as first input
  Product1 : Product  Inputs=*//  SaturateOnIntegerOverflow=on  RndMeth=Zero  InputSameDT=on  OutDataTypeStr=Inherit: Same as first input
  Product3 : Product  Inputs=*//  SaturateOnIntegerOverflow=on  RndMeth=Zero  InputSameDT=on  OutDataTypeStr=Inherit: Same as first input
  Switch : Switch  Threshold=1  SaturateOnIntegerOverflow=on  InputSameDT=on
  mt[kg/sec] : Outport
  forwardmt : Outport  Port=2
  wires:
  Ne[rpm]/1 -> Back-Flow/2(Ne[rpm]), Forward-Flow/3(Ne[rpm])
  Back-Flow/1(mt_dot[kg/s]) -> Gain/1  "rv"
  Product3/1 -> Back-Flow/3(Ro_m)
  Forward-Flow/1(mt_dot[kg/s]) -> forwardmt/1, Switch/1  "ff"
  Tim[K]/1 -> Product3/2
  [Rim] -> Product3/3
  [Ta] -> Product1/2
  [Pa] -> Product1/1
  [Ra] -> Product1/3
  R_im/1 -> [Rim]
  R_a/1 -> [Ra]
  Ta[K]/1 -> [Ta]
  Pa[Pa]/1 -> [Pa]
  Pim[Pa]/1 -> Product3/1, Back-Flow/5(Pm), Product/1, Forward-Flow/5(Pm)
  [Pa] -> Back-Flow/4(Pa), Forward-Flow/4(Pa), Product/2
  TA[deg]/1 -> Back-Flow/1(TA[deg]), Forward-Flow/2(TA[deg])
  Product/1 -> Switch/2  "pr_exhaust_by_intake"
  Switch/1 -> mt[kg/sec]/1
  Product1/1 -> Forward-Flow/1(Ro_a)
  Gain/1 -> Switch/3

== system KD_cl_harness_forthao/ctrl_rb_explicit_20131031_v2/EGR_max_flow/Air_Model_map_use/Forward_Flow ==
  Ro_a : Inport
  Ne_rpm : Inport  Port=2
  Pa : Inport  Port=3
  Pm : Inport  Port=4
  Cal_phi : Subsystem
  Constant2 : Constant  Value=c_p1429  OutDataTypeStr=single
      settings: AttributesFormatString=%<Value>
  Constant3 : Constant  Value=c_1  OutDataTypeStr=single
      settings: AttributesFormatString=%<Value>
  Constant4 : Constant  Value=c_p5401  OutDataTypeStr=single
      settings: AttributesFormatString=%<Value>
  Constant5 : Constant  Value=c_p4167  OutDataTypeStr=single
      settings: AttributesFormatString=%<Value>
  Lookup Table : Lookup  InputValues=invtacols  Table=maxA_t
  Pm_by_Pa : Product  Inputs=*/  SaturateOnIntegerOverflow=on  RndMeth=Zero  InputSameDT=on  OutDataTypeStr=Inherit: Same as first input
  Relational Operator : RelationalOperator  Operator=>  OutDataTypeStr=boolean
      settings: AttributesFormatString=%<Operator>
  Saturation1 : Saturate  UpperLimit=c_1  LowerLimit=c_p4167
      settings: AttributesFormatString=%<UpperLimit>\n%<LowerLimit>
  Saturation2 : Saturate  UpperLimit=c_inf  LowerLimit=c_0
      settings: AttributesFormatString=%<LowerLimit>\n%<UpperLimit>
  Saturation3 : Saturate  UpperLimit=c_inf  LowerLimit=c_100
      settings: AttributesFormatString=%<LowerLimit>\n%<UpperLimit>
  Sqrt : Sqrt  AlgorithmType=Newton-Raphson  SaturateOnIntegerOverflow=on
  Sum : Sum  Inputs=|+-
  Sum1 : Sum  Inputs=|++
  Switch1 : Switch  Criteria=u2 ~= 0
      settings: AttributesFormatString=%<Criteria>
  correct flow1 : Product  Inputs=**  SaturateOnIntegerOverflow=on  RndMeth=Zero  InputSameDT=on  OutDataTypeStr=Inherit: Same as first input
  correct flow2 : Product  Inputs=***  SaturateOnIntegerOverflow=on  RndMeth=Zero  InputSameDT=on  OutDataTypeStr=Inherit: Same as first input
  correct flow3 : Product  Inputs=**  SaturateOnIntegerOverflow=on  RndMeth=Zero  InputSameDT=on  OutDataTypeStr=Inherit: Same as first input
  tokgps1 : Gain  Gain=c_1000inv
  mt_dot_kg_per_s : Outport
  wires:
  Sqrt/1 -> Switch1/1
  correct flow3/1 -> Saturation2/1
  correct flow1/1 -> Sum1/1
  Constant2/1 -> correct flow1/2
  Sum/1 -> correct flow3/1, correct flow1/1
  Constant3/1 -> Sum/1
  Lookup Table/1 -> correct flow2/2  "B_TA"
  Ne_rpm/1 -> Lookup Table/1
  Ro_a/1 -> Cal_phi/2(Ro_a)
  Pa/1 -> [Pa], Saturation3/1
  Pm/1 -> Pm_by_Pa/1
  Pm_by_Pa/1 -> Saturation1/1, Relational Operator/1
  tokgps1/1 -> mt_dot_kg_per_s/1
  correct flow2/1 -> tokgps1/1
  Saturation1/1 -> Sum1/2, Sum/2
  Switch1/1 -> correct flow2/3
  Cal_phi/1(phi) -> correct flow2/1
  Sum1/1 -> correct flow3/2
  [Pa] -> Cal_phi/1(Pa)
  Saturation2/1 -> Sqrt/1
  Saturation3/1 -> Pm_by_Pa/2
  Relational Operator/1 -> Switch1/2
  Constant4/1 -> Switch1/3
  Constant5/1 -> Relational Operator/2

== system KD_cl_harness_forthao/ctrl_rb_explicit_20131031_v2/While_Iterator_Subsystem/newton/For_Iterator_Subsystem ==
  u : Inport
  sv1 : Inport  Port=2
  sv2 : Inport  Port=3
  arg : Inport  Port=4
  beta : Inport  Port=5
  Demux : Demux  Outputs=2
  Divide : Product  Inputs=*/
  For Iterator : ForIterator  ResetStates=reset  IterationLimit=SVR_EGR_exhat.num_SV
  Gain : Gain  Gain=100
      settings: AttributesFormatString=%<Gain>
  Product{,1..3} (4 alike) : Product  RndMeth=Zero
  Saturation1 : Saturate  UpperLimit=9  LowerLimit=1
      settings: AttributesFormatString=%<LowerLimit>\n%<UpperLimit>
  Selector : Selector  InputPortWidth=SVR_EGR_exhat.num_SV  IndexOptions=Index vector (port)  Indices=[1 3]
  Selector1 : Selector  InputPortWidth=SVR_EGR_exhat.num_SV  IndexOptions=Index vector (port)  Indices=[1 3]
  Selector2 : Selector  InputPortWidth=SVR_EGR_exhat.num_SV  IndexOptions=Index vector (port)  Indices=[1 3]
  Sum : Sum  Inputs=|-+
  Sum1 : Sum  Inputs=+-|
  Sum2 : Sum  Inputs=-|-
  Sum3 : Sum  Inputs=++|
  Unit Delay : UnitDelay  SampleTime=-1
  exp Lookup Table : Lookup  InputValues=SVR_EGR_exhat.exp.x  Table=SVR_EGR_exhat.exp.y  LookUpMeth=Interpolation-Use End Values
      settings: AttributesFormatString=%<LookUpMeth>\n%<InputValues>
  ba : Outport  OutDataTypeStr=single
  wires:
  Saturation1/1 -> [iter]
  For Iterator/1 -> Saturation1/1
  [iter] -> Selector2/2
  [iter] -> Selector1/2
  [iter] -> Selector/2
  Sum3/1 -> ba/1, Unit Delay/1
  Product3/1 -> Sum3/2
  Selector2/1 -> Product3/2
  Gain/1 -> Divide/2
  Product2/1 -> Gain/1
  arg/1 -> Product2/2, Product2/1
  Sum2/1 -> Divide/1
  Product1/1 -> Sum2/2
  Product/1 -> Sum2/1
  Sum1/1 -> Product1/2, Product1/1
  Sum/1 -> Product/2, Product/1
  Demux/2 -> Sum1/1
  Selector1/1 -> Sum1/2
  Demux/1 -> Sum/2
  Selector/1 -> Sum/1
  u/1 -> Demux/1
  beta/1 -> Selector2/1
  sv2/1 -> Selector1/1
  sv1/1 -> Selector/1
  Unit Delay/1 -> Sum3/1
  Divide/1 -> exp Lookup Table/1
  exp Lookup Table/1 -> Product3/1

== system KD_cl_harness_forthao/ctrl_rb_explicit_20131031_v2/While_Iterator_Subsystem/newton/If_Action_Subsystem ==
  pex : Inport
  ba : Inport  Port=2
  c : Inport  Port=3
  k : Inport  Port=4
  Action Port : ActionPort  ActionType=then
  Gain1 : Gain  Gain=2
  Gain6 : Gain  Gain=2
  Mux : Mux  Inputs=2
  Product : Product  Inputs=***  RndMeth=Zero
  Product1 : Product  Inputs=*/  RndMeth=Zero
  Product2 : Product  Inputs=**  RndMeth=Zero
  Product3 : Product  Inputs=***  RndMeth=Zero
  Product4 : Product  Inputs=*/  RndMeth=Zero
  Saturation1 : Saturate  UpperLimit=inf  LowerLimit=0
      settings: AttributesFormatString=%<LowerLimit>\n%<UpperLimit>
  Saturation2 : Saturate  UpperLimit=inf  LowerLimit=0
      settings: AttributesFormatString=%<LowerLimit>\n%<UpperLimit>
  Saturation3 : Saturate  UpperLimit=c_inf  LowerLimit=c_p1e9
      settings: AttributesFormatString=%<LowerLimit>\n%<UpperLimit>
  Saturation4 : Saturate  UpperLimit=c_inf  LowerLimit=c_p1e9
      settings: AttributesFormatString=%<LowerLimit>\n%<UpperLimit>
  Sqrt1 : Sqrt  AlgorithmType=Newton-Raphson  SaturateOnIntegerOverflow=on
  Sqrt2 : Sqrt  AlgorithmType=Newton-Raphson  SaturateOnIntegerOverflow=on
  Sum1 : Sum  Inputs=++|
  Sum3 : Sum  Inputs=++|
  one : Constant  OutDataTypeStr=single  SampleTime=-1
      settings: AttributesFormatString=%<Value>\n%<SampleTime>
  one1 : Constant  OutDataTypeStr=single  SampleTime=-1
      settings: AttributesFormatString=%<Value>\n%<SampleTime>
  Out : Outport
  wires:
  Saturation4/1 -> Product4/2
  Saturation3/1 -> Product1/2
  Saturation2/1 -> Sqrt1/1
  Saturation1/1 -> Sqrt2/1
  Product3/1 -> Product2/1
  Sqrt1/1 -> Product3/3
  Product4/1 -> Saturation2/1
  Gain1/1 -> Saturation4/1
  Sum1/1 -> Gain1/1
  one1/1 -> Sum1/1
  [k] -> Sum1/2
  [k] -> Product4/1
  [c] -> Product3/2
  [ba] -> Product3/1
  Mux/1 -> Out/1
  Product2/1 -> Mux/2
  Product/1 -> Mux/1
  Sqrt2/1 -> Product/3
  [pex] -> Product2/2
  Product1/1 -> Saturation1/1
  Gain6/1 -> Saturation3/1
  Sum3/1 -> Gain6/1
  one/1 -> Sum3/1
  [k] -> Sum3/2
  [k] -> Product1/1
  [c] -> Product/2
  [ba] -> Product/1
  k/1 -> [k]
  pex/1 -> [pex]
  c/1 -> [c]
  ba/1 -> [ba]

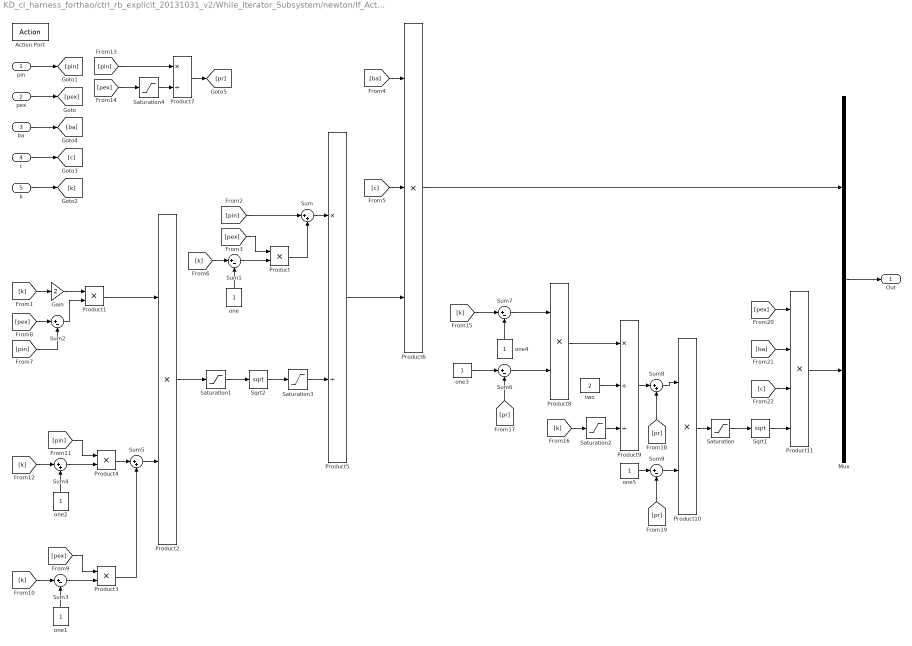
== system KD_cl_harness_forthao/ctrl_rb_explicit_20131031_v2/While_Iterator_Subsystem/newton/If_Action_Subsystem1 ==
  pin : Inport
  pex : Inport  Port=2
  ba : Inport  Port=3
  c : Inport  Port=4
  k : Inport  Port=5
  Action Port : ActionPort  ActionType=else
  Gain : Gain  Gain=2
  Mux : Mux  Inputs=2
  Product{,1..4} (5 alike) : Product  RndMeth=Zero
  Product10 : Product  Inputs=**  RndMeth=Zero
  Product11 : Product  Inputs=****  RndMeth=Zero
  Product5 : Product  Inputs=*/  RndMeth=Zero
  Product6 : Product  Inputs=***  RndMeth=Zero
  Product7 : Product  Inputs=*/  RndMeth=Zero
  Product8 : Product  Inputs=**  RndMeth=Zero
  Product9 : Product  Inputs=*//  RndMeth=Zero
  Saturation : Saturate  UpperLimit=inf  LowerLimit=0
      settings: AttributesFormatString=%<LowerLimit>\n%<UpperLimit>
  Saturation1 : Saturate  UpperLimit=inf  LowerLimit=0
      settings: AttributesFormatString=%<LowerLimit>\n%<UpperLimit>
  Saturation2 : Saturate  UpperLimit=c_inf  LowerLimit=c_p1e9
      settings: AttributesFormatString=%<LowerLimit>\n%<UpperLimit>
  Saturation3 : Saturate  UpperLimit=c_inf  LowerLimit=c_p00001
      settings: AttributesFormatString=%<LowerLimit>\n%<UpperLimit>
  Saturation4 : Saturate  UpperLimit=c_inf  LowerLimit=c_p1e9
      settings: AttributesFormatString=%<LowerLimit>\n%<UpperLimit>
  Sqrt1 : Sqrt  AlgorithmType=Newton-Raphson  SaturateOnIntegerOverflow=on
  Sqrt2 : Sqrt  AlgorithmType=Newton-Raphson  SaturateOnIntegerOverflow=on
  Sum{,4..5,8} (4 alike) : Sum  Inputs=|++
  Sum{1..3,6..7,9} (6 alike) : Sum  Inputs=|+-
  one{,1..5} (6 alike) : Constant  OutDataTypeStr=single  SampleTime=-1
      settings: AttributesFormatString=%<Value>\n%<SampleTime>
  two : Constant  Value=2  OutDataTypeStr=single  SampleTime=-1
      settings: AttributesFormatString=%<Value>\n%<SampleTime>
  Out : Outport
  wires:
  Saturation4/1 -> Product7/2
  Saturation2/1 -> Product9/3
  Saturation1/1 -> Sqrt2/1
  Saturation/1 -> Sqrt1/1
  Mux/1 -> Out/1
  Product6/1 -> Mux/1
  Product11/1 -> Mux/2
  [c] -> Product11/3
  [ba] -> Product11/2
  [pex] -> Product11/1
  Sqrt1/1 -> Product11/4
  Product10/1 -> Saturation/1
  Sum8/1 -> Product10/1
  [pr] -> Sum9/2
  Sum9/1 -> Product10/2
  one5/1 -> Sum9/1
  [pr] -> Sum8/2
  Product9/1 -> Sum8/1
  [pr] -> Sum6/2
  Product7/1 -> [pr]
  [k] -> Saturation2/1
  two/1 -> Product9/2
  Product8/1 -> Product9/1
  Sum7/1 -> Product8/1
  Sum6/1 -> Product8/2
  one4/1 -> Sum7/2
  [k] -> Sum7/1
  [pex] -> Saturation4/1
  [pin] -> Product7/1
  one3/1 -> Sum6/1
  Product5/1 -> Product6/3
  [c] -> Product6/2
  [ba] -> Product6/1
  Sum/1 -> Product5/1
  Sqrt2/1 -> Saturation3/1
  Product2/1 -> Saturation1/1
  Product3/1 -> Sum5/2
  Product4/1 -> Sum5/1
  Sum5/1 -> Product2/2
  [pin] -> Product4/1
  Sum4/1 -> Product4/2
  [k] -> Sum4/1
  one2/1 -> Sum4/2
  [pex] -> Product3/1
  Sum3/1 -> Product3/2
  [k] -> Sum3/1
  one1/1 -> Sum3/2
  Product1/1 -> Product2/1
  Gain/1 -> Product1/1
  Sum2/1 -> Product1/2
  [pex] -> Sum2/1
  [pin] -> Sum2/2
  [k] -> Gain/1
  Product/1 -> Sum/2
  [pex] -> Product/1
  Sum1/1 -> Product/2
  [k] -> Sum1/1
  one/1 -> Sum1/2
  [pin] -> Sum/1
  pin/1 -> [pin]
  k/1 -> [k]
  c/1 -> [c]
  ba/1 -> [ba]
  pex/1 -> [pex]
  Saturation3/1 -> Product5/2

== system KD_cl_harness_forthao/ctrl_rb_explicit_20131031_v2/While_Iterator_Subsystem/newton/If_Action_Subsystem2 ==
  pex_hat : Inport
  Action Port : ActionPort  ActionType=else
  pex : Outport
  wires:
  pex_hat/1 -> pex/1

== system KD_cl_harness_forthao/ctrl_rb_explicit_20131031_v2/While_Iterator_Subsystem/newton/If_Action_Subsystem3 ==
  valve : Inport
  pex_hat : Inport  Port=2
  pex_ecu : Inport  Port=3
  Action Port : ActionPort  ActionType=then
  Divide : Product  Inputs=*/
  Divide1 : Product  Inputs=**
  Divide2 : Product  Inputs=**
  Sum : Sum  Inputs=-+|
  Sum1 : Sum  Inputs=+|+
  fifteen : Constant  Value=15  OutDataTypeStr=single
      settings: AttributesFormatString=%<Value>
  one : Constant  OutDataTypeStr=single
      settings: AttributesFormatString=%<Value>
  pex : Outport
  wires:
  valve/1 -> Divide/1
  fifteen/1 -> Divide/2
  Divide/1 -> Divide1/2, Sum/1
  pex_hat/1 -> Divide1/1
  one/1 -> Sum/2
  Sum/1 -> Divide2/1
  pex_ecu/1 -> Divide2/2
  Divide1/1 -> Sum1/1
  Divide2/1 -> Sum1/2
  Sum1/1 -> pex/1

== system KD_cl_harness_forthao/ctrl_rb_explicit_20131031_v2/While_Iterator_Subsystem/newton/update ==
  dwdp : Inport
  error : Inport  Port=2
  Data Store Read1 : DataStoreRead  DataStoreName=man_pex_eps
  Data Store Read11 : DataStoreRead  DataStoreName=man_pex_eps
  Data Store Read16 : DataStoreRead  DataStoreName=man_use_LM
  Product2 : Product  Inputs=**  RndMeth=Zero
  Product3 : Product  Inputs=/*  RndMeth=Zero
  Product8 : Product  Inputs=/**  RndMeth=Zero
  Relational Operator7 : RelationalOperator  Operator=>  OutDataTypeStr=boolean
      settings: AttributesFormatString=%<Operator>
  Saturation1 : Saturate  UpperLimit=c_inf  LowerLimit=c_p1e9
      settings: AttributesFormatString=%<LowerLimit>\n%<UpperLimit>
  Saturation3 : Saturate  UpperLimit=c_inf  LowerLimit=c_p1e9
      settings: AttributesFormatString=%<LowerLimit>\n%<UpperLimit>
  Sum1 : Sum  Inputs=|++
  Sum2 : Sum  Inputs=|++
  Switch7 : Switch  Criteria=u2 ~= 0
      settings: AttributesFormatString=%<Criteria>
  man_pex_eps : Gain
  man_pex_eps1 : Gain
  man_use_LM : Gain
  zero8 : Constant  Value=0  OutDataTypeStr=single  SampleTime=-1
      settings: AttributesFormatString=%<Value>\n%<SampleTime>
  delta : Outport
  wires:
  Data Store Read11/1 -> man_pex_eps/1
  Sum2/1 -> Saturation3/1
  Saturation3/1 -> Product8/1
  Product2/1 -> Sum2/2
  error/1 -> [e]
  dwdp/1 -> [dwdp]
  [dwdp] -> Product2/1, Product8/2, Product2/2
  [e] -> Product8/3
  Data Store Read1/1 -> man_pex_eps1/1
  Sum1/1 -> Saturation1/1
  Saturation1/1 -> Product3/1
  [dwdp] -> Sum1/2
  [e] -> Product3/2
  zero8/1 -> Relational Operator7/2
  Data Store Read16/1 -> man_use_LM/1
  Relational Operator7/1 -> Switch7/2
  Product3/1 -> Switch7/3
  Product8/1 -> Switch7/1
  Switch7/1 -> delta/1
  man_pex_eps/1 -> Sum2/1
  man_pex_eps1/1 -> Sum1/1
  man_use_LM/1 -> Relational Operator7/1
